simulink model "FluidSimWithoutController_v2_2018a"  (R2018a)
settings: Solver=VariableStepAuto  StartTime=0.0  StopTime=100  RelTol=1e-3
libraries: fl_lib x12, nesl_utility x6, sh_lib x5, simulink x1
settings Model: Creator=Simon  LastModifiedBy=mkell

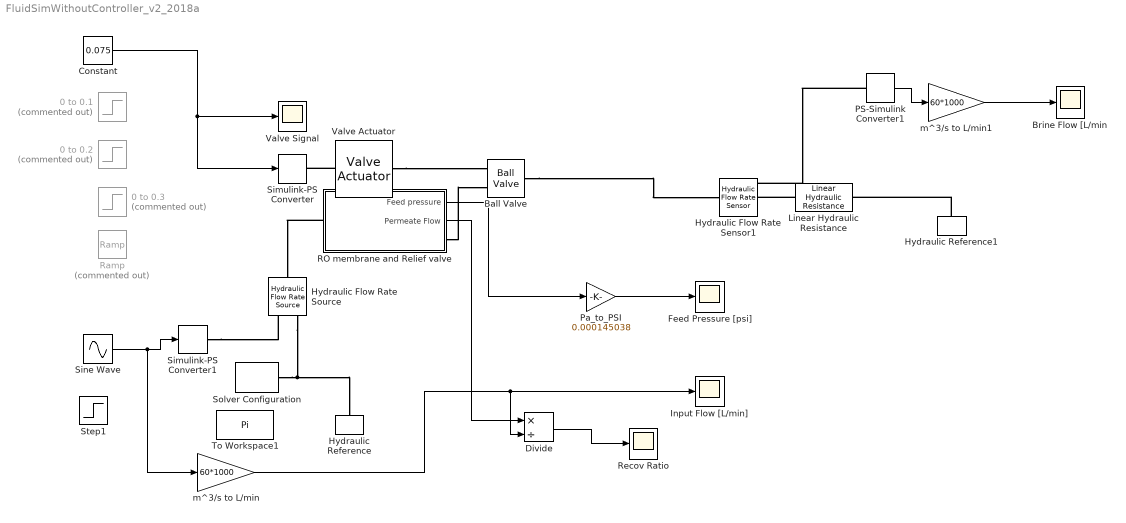
== system FluidSimWithoutController_v2_2018a ==
  0 to 0.1 : Step  Commented=on  Time=10  After=0.1  SampleTime=0
  0 to 0.2 : Step  Commented=on  Time=10  After=0.2  SampleTime=0
  0 to 0.3 : Step  Commented=on  Time=3  After=0.05*1.5  SampleTime=0
  Ball Valve : sh_lib/Valves/Flow Control Valves/Ball Valve  valve_seat_spec=1  cone_ang=120 deg  d_ball=0.01 m  d_orif=5e-3 m  x_0=0 m  C_d=0.65  A_leak=1e-12 m^2  lam_spec=1  B_lam=0.999  Re_cr=10  flow_rate_specify=off  flow_rate_priority=None  flow_rate=0.001 m^3/s  flow_rate_nominal_specify=off  flow_rate_nominal_unit=m^3/s  flow_rate_nominal_value=1  pressure_drop_specify=off  pressure_drop_priority=None  pressure_drop=0 Pa  pressure_drop_nominal_specify=off  pressure_drop_nominal_unit=Pa  pressure_drop_nominal_value=1
      settings: SourceProductBaseCode=SH  InternalSimscapePortConfiguration="{\"Bottom\":[],\"Left\":[{\"id\":\"S\",\"label\":\"S\",\"type\":\"input\"},{\"id\":\"A\",\"label\":\"A\",\"type\":\"foundation.hydraulic.hydraulic\"}],\"Right\":[{\"id\":\"B\",\"label\":\"B\",\"type\":\"foundation.hydraulic.hydraulic\"}],\"Top\":[]}"
  Brine Flow [L/min : Scope
  Constant : Constant  Value=0.075  SampleTime=0
  Divide : Product  Inputs=*/
  Feed Pressure [psi] : Scope
  Hydraulic Flow Rate Sensor1 : fl_lib/Hydraulic/Hydraulic Sensors/Hydraulic Flow Rate Sensor
  Hydraulic Flow Rate Source : fl_lib/Hydraulic/Hydraulic Sources/Hydraulic Flow Rate Source
      settings: SourceProductBaseCode=SS  InternalSimscapePortConfiguration="{\"Bottom\":[],\"Left\":[{\"id\":\"P\",\"label\":\"P\",\"type\":\"foundation.hydraulic.hydraulic\"}],\"Right\":[{\"id\":\"S\",\"label\":\"S\",\"type\":\"input\"},{\"id\":\"T\",\"label\":\"T\",\"type\":\"foundation.hydraulic.hydraulic\"}],\"Top\":[]}"
  Hydraulic Reference : fl_lib/Hydraulic/Hydraulic Elements/Hydraulic Reference
  Hydraulic Reference1 : fl_lib/Hydraulic/Hydraulic Elements/Hydraulic Reference
  Input Flow [L/min] : Scope
  Linear Hydraulic Resistance : fl_lib/Hydraulic/Hydraulic Elements/Linear Hydraulic Resistance  resistance=1 Pa/(m^3/s)  q_specify=off  q_priority=None  q=0.001 m^3/s  q_nominal_specify=off  q_nominal_unit=m^3/s  q_nominal_value=1  p_specify=off  p_priority=None  p=0 Pa  p_nominal_specify=off  p_nominal_unit=Pa  p_nominal_value=1
      settings: SourceProductBaseCode=SS  InternalSimscapePortConfiguration="{\"Bottom\":[],\"Left\":[{\"id\":\"A\",\"label\":\"A\",\"type\":\"foundation.hydraulic.hydraulic\"}],\"Right\":[{\"id\":\"B\",\"label\":\"B\",\"type\":\"foundation.hydraulic.hydraulic\"}],\"Top\":[]}"
  PS-Simulink Converter1 : nesl_utility/PS-Simulink Converter  PhysicalDomain=network_engine_domain  SubClassName=ps_output  LeftPortType=input  RightPortType=output  PseudoPeriodic=off  Frequencies=[]  Unit=1  AffineConversion=off
  Pa_to_PSI : Gain  Gain=0.000145038
  RO membrane and Relief valve : Subsystem
  Ramp : simulink/Sources/Ramp  Commented=on  slope=0.005*2  start=0  InitialOutput=0
  "Recov Ratio " : Scope
  Simulink-PS Converter : nesl_utility/Simulink-PS Converter  PhysicalDomain=network_engine_domain  SubClassName=ps_input  LeftPortType=input  RightPortType=output  PseudoPeriodic=off  Frequencies=[]  NoiseDistribution=none  NoiseParameters=[]  Unit=1  AffineConversion=off  FilteringAndDerivatives=provide  SimscapeFilterOrder=1  InputFilterTimeConstant=0.001  UdotUserProvided=0
  Simulink-PS Converter1 : nesl_utility/Simulink-PS Converter  PhysicalDomain=network_engine_domain  SubClassName=ps_input  LeftPortType=input  RightPortType=output  PseudoPeriodic=off  Frequencies=[]  NoiseDistribution=none  NoiseParameters=[]  Unit=m^3/s  AffineConversion=off  FilteringAndDerivatives=provide  SimscapeFilterOrder=1  InputFilterTimeConstant=0.001  UdotUserProvided=0
  Sine Wave : Sin  Amplitude=3/1000/60  Bias=5/1000/60  Frequency=2*pi/8  SampleTime=0
  Solver Configuration : nesl_utility/Solver Configuration  PhysicalDomain=network_engine_domain  SubClassName=solver  LeftPortType=input  RightPortType=generic  Tones=[]  Harmonics=[]  SimulateNoise=off  Profile=off  UseLocalSampling=off  EnableSwitchedLinearOptims=on  FrequencyDomain=off  UseCCode=off  RelTol=0.001  AbsTol=1e-06  MinStep=1e-09  ToWorkspace=off  RevertToSquareIcSolve=off  NumHomotopyIterations=100  PhasorMode=off  PhasorModeNumHarmonics=1  DoDC=off  ResidualTolerance=1e-09  UseLocalSolver=off  LocalSolverChoice=NE_BACKWARD_EULER_ADVANCER  LocalSolverSampleTime=0.001  DoFixedCost=off  MaxNonlinIter=3  MaxModeIter=2  ComputeImpulses=off  ImpulseIterations=2  LinearAlgebra=Sparse  EquationFormulation=NE_TIME_EF  DelaysMemoryBudget=1024  AutomaticFiltering=on  FilteringTimeConstant=0.001  PartitionStorageMethod=AS_NEEDED  PartitionMemoryBudget=1024  PartitionMethod=FAST
  Step1 : Step  Before=0.001/1000/60  After=2.5/1000/60  SampleTime=0
  To Workspace1 : ToWorkspace  VariableName=Pi  SaveFormat=Timeseries  SampleTime=-1
  Valve Actuator : sh_lib/Valves/Valve Actuators/Valve Actuator  valve_stroke=0.005 m  time_constant=10 s  gain=5e-4 m
      settings: SourceProductBaseCode=SH  InternalSimscapePortConfiguration="{\"Bottom\":[],\"Left\":[{\"id\":\"I\",\"label\":\"\",\"type\":\"input\"}],\"Right\":[{\"id\":\"O\",\"label\":\"\",\"type\":\"output\"}],\"Top\":[]}"
  Valve Signal : Scope
  m^3/s to L/min : Gain  Gain=60*1000
  m^3/s to L/min1 : Gain  Gain=60*1000
  wires:
  RO membrane and Relief valve/1(Feed pressure) -> Pa_to_PSI/1
  m^3/s to L/min/1 -> Divide/2, Input Flow [L/min]/1
  Pa_to_PSI/1 -> Feed Pressure [psi]/1
  RO membrane and Relief valve/2(Permeate Flow) -> Divide/1
  Divide/1 -> "Recov Ratio "/1
  Constant/1 -> Valve Signal/1, Simulink-PS Converter/1
  Sine Wave/1 -> m^3/s to L/min/1, Simulink-PS Converter1/1
  m^3/s to L/min1/1 -> Brine Flow [L/min/1
  PS-Simulink Converter1/1 -> m^3/s to L/min1/1
  connections:
  Solver Configuration/RConn1 -- Hydraulic Flow Rate Source/RConn2 -- Hydraulic Reference/LConn1
  PS-Simulink Converter1/LConn1 -- Hydraulic Flow Rate Sensor1/RConn1
  Valve Actuator/LConn1 -- Simulink-PS Converter/RConn1
  Ball Valve/RConn1 -- Hydraulic Flow Rate Sensor1/LConn1
  Valve Actuator/RConn1 -- Ball Valve/LConn1
  Simulink-PS Converter1/RConn1 -- Hydraulic Flow Rate Source/RConn1
  Hydraulic Reference1/LConn1 -- Linear Hydraulic Resistance/RConn1
  RO membrane and Relief valve/LConn1 -- Hydraulic Flow Rate Source/LConn1
  RO membrane and Relief valve/RConn1 -- Ball Valve/LConn2
  Linear Hydraulic Resistance/LConn1 -- Hydraulic Flow Rate Sensor1/RConn2

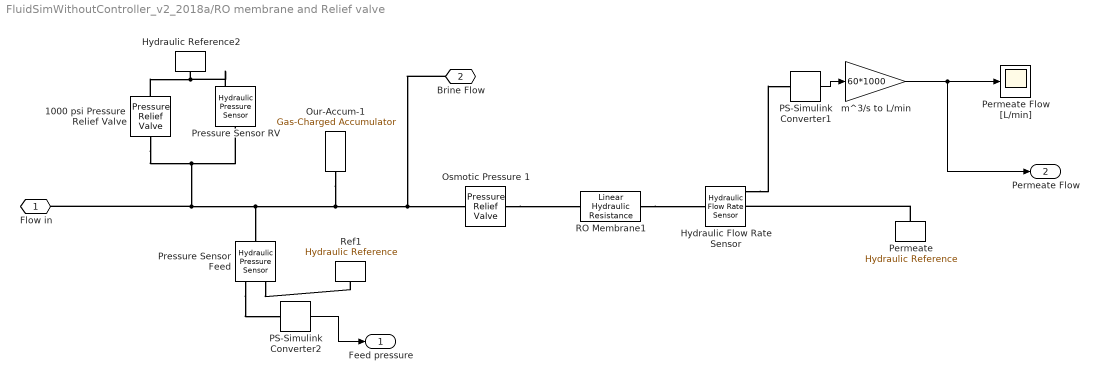
== system FluidSimWithoutController_v2_2018a/RO membrane and Relief valve ==
  1000 psi Pressure Relief Valve : sh_lib/Valves/Pressure Control Valves/Pressure Relief Valve  valve_area_spec=1  p_diff_TLU=[30.15e5 : 15e3 : 31.35e5] Pa  area_TLU=[1 : 1 : 9] .* 1e-5 m^2  area_max=pi*(0.75/2)^2 in^2  pres_set=1000 psi  reg_range=50 psi  C_d=0.7  A_leak=1e-12 m^2  lam_spec=1  B_lam=0.999  Re_cr=12  dynamic=0  tau=0.1 s  area_init=1e-12 m^2
      settings: SourceProductBaseCode=SH  InternalSimscapePortConfiguration="{\"Bottom\":[],\"Left\":[{\"id\":\"A\",\"label\":\"A\",\"type\":\"foundation.hydraulic.hydraulic\"}],\"Right\":[{\"id\":\"B\",\"label\":\"B\",\"type\":\"foundation.hydraulic.hydraulic\"}],\"Top\":[]}"
  Hydraulic Flow Rate Sensor : fl_lib/Hydraulic/Hydraulic Sensors/Hydraulic Flow Rate Sensor
  Hydraulic Reference2 : fl_lib/Hydraulic/Hydraulic Elements/Hydraulic Reference
  Osmotic Pressure 1 : sh_lib/Valves/Pressure Control Valves/Pressure Relief Valve  valve_area_spec=1  p_diff_TLU=[30.15e5 : 15e3 : 31.35e5] Pa  area_TLU=[1 : 1 : 9] .* 1e-5 m^2  area_max=10*pi*(0.75/2)^2 in^2  pres_set=30 bar  reg_range=2 bar  C_d=0.7  A_leak=1e-12 m^2  lam_spec=1  B_lam=0.999  Re_cr=12  dynamic=0  tau=0.1 s  area_init=1e-12 m^2
      settings: SourceProductBaseCode=SH  InternalSimscapePortConfiguration="{\"Bottom\":[],\"Left\":[{\"id\":\"A\",\"label\":\"A\",\"type\":\"foundation.hydraulic.hydraulic\"}],\"Right\":[{\"id\":\"B\",\"label\":\"B\",\"type\":\"foundation.hydraulic.hydraulic\"}],\"Top\":[]}"
  Our-Accum-1 : sh_lib/Accumulators/Gas-Charged Accumulator  capacity=accumulator_volume l  dead_volume=minimum_gas_volume l  pr_preload=precharge_pressure Pa  k_sh=1.4  stiff_coeff=1e7 Pa/m^3  penetr_coeff=1e7 s*Pa/m^6  flow_rate_specify=on  flow_rate_priority=None  flow_rate=0 m^3/s  flow_rate_nominal_specify=off  flow_rate_nominal_unit=m^3/s  flow_rate_nominal_value=1  liquid_volume_specify=on  liquid_volume_priority=High  liquid_volume=0 m^3  liquid_volume_nominal_specify=off  liquid_volume_nominal_unit=m^3  liquid_volume_nominal_value=1  liquid_pressure_specify=off  liquid_pressure_priority=None  liquid_pressure=1.01325e+5 Pa  liquid_pressure_nominal_specify=off  liquid_pressure_nominal_unit=Pa  liquid_pressure_nominal_value=1
      settings: SourceProductBaseCode=SH  InternalSimscapePortConfiguration="{\"Bottom\":[],\"Left\":[],\"Right\":[{\"id\":\"A\",\"label\":\"A\",\"type\":\"foundation.hydraulic.hydraulic\"}],\"Top\":[]}"
  PS-Simulink Converter1 : nesl_utility/PS-Simulink Converter  PhysicalDomain=network_engine_domain  SubClassName=ps_output  LeftPortType=input  RightPortType=output  PseudoPeriodic=off  Frequencies=[]  Unit=m^3/s  AffineConversion=off
  PS-Simulink Converter2 : nesl_utility/PS-Simulink Converter  PhysicalDomain=network_engine_domain  SubClassName=ps_output  LeftPortType=input  RightPortType=output  PseudoPeriodic=off  Frequencies=[]  Unit=Pa  AffineConversion=off
  Permeate : fl_lib/Hydraulic/Hydraulic Elements/Hydraulic Reference
  Permeate Flow [L/min] : Scope
  Pressure Sensor RV : fl_lib/Hydraulic/Hydraulic Sensors/Hydraulic Pressure Sensor
  Pressure Sensor Feed : fl_lib/Hydraulic/Hydraulic Sensors/Hydraulic Pressure Sensor
  RO Membrane1 : fl_lib/Hydraulic/Hydraulic Elements/Linear Hydraulic Resistance  resistance=35449930518.1362 Pa/(m^3/s)  q_specify=off  q_priority=None  q=0.001 m^3/s  q_nominal_specify=off  q_nominal_unit=m^3/s  q_nominal_value=1  p_specify=off  p_priority=None  p=0 Pa  p_nominal_specify=off  p_nominal_unit=Pa  p_nominal_value=1
      settings: SourceProductBaseCode=SS  InternalSimscapePortConfiguration="{\"Bottom\":[],\"Left\":[{\"id\":\"A\",\"label\":\"A\",\"type\":\"foundation.hydraulic.hydraulic\"}],\"Right\":[{\"id\":\"B\",\"label\":\"B\",\"type\":\"foundation.hydraulic.hydraulic\"}],\"Top\":[]}"
  Ref1 : fl_lib/Hydraulic/Hydraulic Elements/Hydraulic Reference
  m^3/s to L/min : Gain  Gain=60*1000
  Flow in : PMIOPort  Side=Left
  Brine Flow : PMIOPort  Port=2  Side=Right
  Feed pressure : Outport
  Permeate Flow : Outport  Port=2
  wires:
  PS-Simulink Converter2/1 -> Feed pressure/1
  m^3/s to L/min/1 -> Permeate Flow [L/min]/1, Permeate Flow/1
  PS-Simulink Converter1/1 -> m^3/s to L/min/1
  connections:
  1000 psi Pressure Relief Valve/LConn1 -- Pressure Sensor RV/LConn1 -- Flow in/RConn1 -- Our-Accum-1/RConn1 -- Brine Flow/RConn1 -- Osmotic Pressure 1/LConn1 -- Pressure Sensor Feed/LConn1
  Pressure Sensor RV/RConn1 -- Hydraulic Reference2/LConn1 -- 1000 psi Pressure Relief Valve/RConn1
  Osmotic Pressure 1/RConn1 -- RO Membrane1/LConn1
  Pressure Sensor Feed/RConn1 -- Ref1/LConn1
  Pressure Sensor Feed/RConn2 -- PS-Simulink Converter2/LConn1
  RO Membrane1/RConn1 -- Hydraulic Flow Rate Sensor/LConn1
  Permeate/LConn1 -- Hydraulic Flow Rate Sensor/RConn2
  Hydraulic Flow Rate Sensor/RConn1 -- PS-Simulink Converter1/LConn1
